simulink model "SerialTest"  (R2014a)
settings: Solver=FixedStepDiscrete  StartTime=0.0  StopTime=inf  FixedStep=0.1  RelTol=1e-3
settings Model: SimulationMode=external  ExtModeTrigDuration=100  Creator=omcaree  LastModifiedBy=omcaree
settings OptimizationCC: OptimizeModelRefInitCode=on  LifeSpan=1
settings DebuggingCC: UnderspecifiedInitializationDetection=Classic  SolverPrmCheckMsg=none
settings HardwareCC: ProdLargestAtomicInteger=Long  ProdLargestAtomicFloat=Double  ProdEndianess=LittleEndian  ProdHWDeviceType=ARM Compatible->ARM Cortex
settings RTWCC: SystemTargetFile=realtime.tlc  GenerateMakefile=off  TemplateMakefile=realtime.tmf  Description=Run on Target Hardware  RTWVerbose=off  ProcessScript=realtime_make_rtw_hook  CustomSource=SerialPort.c
settings STFCustomTargetCC: TargetLibSuffix=.a  GenerateSampleERTMain=on  ConcurrentExecutionCompliant=off  GeneratePreprocessorConditionals=Use local settings  ERTCustomFileBanners=on  SupportNonInlinedSFcns=off  SupportVariableSizeSignals=on  MATLABClassNameForMDSCustomization=Simulink.SoftwareTarget.ERTCustomization  GRTInterface=off  SystemTargetFile=realtime.tlc
settings ERTTargetCC: CombineOutputUpdateFcns=off  SupportContinuousTime=on  SupportVariableSizeSignals=on  ExtMode=on  ExtModeMexArgs='169.254.0.31' 0 17725 30  ERTSrcFileBannerTemplate=realtime_code_template.cgt  ERTHdrFileBannerTemplate=realtime_code_template.cgt  ERTDataSrcFileTemplate=realtime_code_template.cgt  ERTDataHdrFileTemplate=realtime_code_template.cgt  ERTCustomFileTemplate=realtime_file_process.tlc

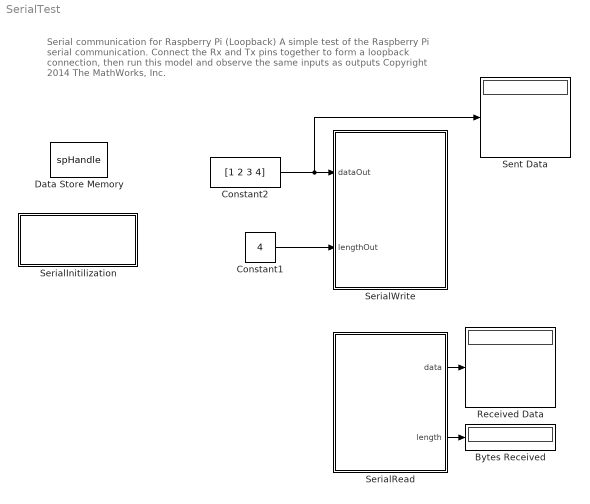
== system SerialTest ==
  note: Serial communication for Raspberry Pi (Loopback)
      |
      | A simple test of the Raspberry Pi serial communication. Connect the Rx and Tx pins together to form a
      | loopback connection, then run this model and observe the same inputs as outputs
      |
      | Copyright 2014 The MathWorks, Inc.
  Bytes Received : Display
  Constant1 : Constant  Value=4
  Constant2 : Constant  Value=[1 2 3 4]  OutDataTypeStr=uint8
  Data Store Memory : DataStoreMemory  DataStoreName=spHandle  ReadBeforeWriteMsg=warning  WriteAfterWriteMsg=warning  WriteAfterReadMsg=warning  InitialValue=-1  OutDataTypeStr=int32
  Received Data : Display
  Sent Data : Display
  SerialInitilization : MATLAB Function  TreatAsAtomicUnit=on
  SerialRead : MATLAB Function  TreatAsAtomicUnit=on
  SerialWrite : MATLAB Function  TreatAsAtomicUnit=on
  wires:
  SerialRead/2(length) -> Bytes Received/1
  Constant1/1 -> SerialWrite/2(lengthOut)
  Constant2/1 -> Sent Data/1, SerialWrite/1(dataOut)
  SerialRead/1(data) -> Received Data/1

== matlab function SerialTest/SerialInitilization ==
  data: spHandle data_store_memory
function initSerial
global spHandle;
if ~coder.target('SFun')   
    if isempty(spHandle)||spHandle==-1;
        spHandle=int32(0);
        spHandle =coder.ceval('setupSerialPort',['/dev/ttyAMA0' 0], uint32(57600));
    end 
end

== matlab function SerialTest/SerialRead ==
  data: data output; length output; spHandle data_store_memory
function [data,length]=serialRead
global spHandle;
data = zeros(512,1,'uint8');
length =int32(0);
if ~coder.target('SFun')
    if spHandle>0
        bytesRead = int32(0);
        dataRead = zeros(512,1,'uint8');
        bytesRead = coder.ceval('read',spHandle, coder.ref(dataRead), uint32(512));
        if bytesRead>0
            data= dataRead;
            length=bytesRead;
        end
    end
end

== matlab function SerialTest/SerialWrite ==
  data: dataOut input uint8; lengthOut input; spHandle data_store_memory
function serialWrite(dataOut, lengthOut)
global spHandle;
if ~coder.target('SFun')  
        if lengthOut>0           
            coder.ceval('write',spHandle, coder.ref(dataOut), uint32(lengthOut));
        end   
end
